simulink model "exp1_2"  (R2019a)
settings: Solver=VariableStepAuto  StartTime=0.0  StopTime=10.0  RelTol=1e-3
undefined symbols (not defined in the file or in its folder): sfunchk
settings Model: Creator=17827  LastModifiedBy=17827

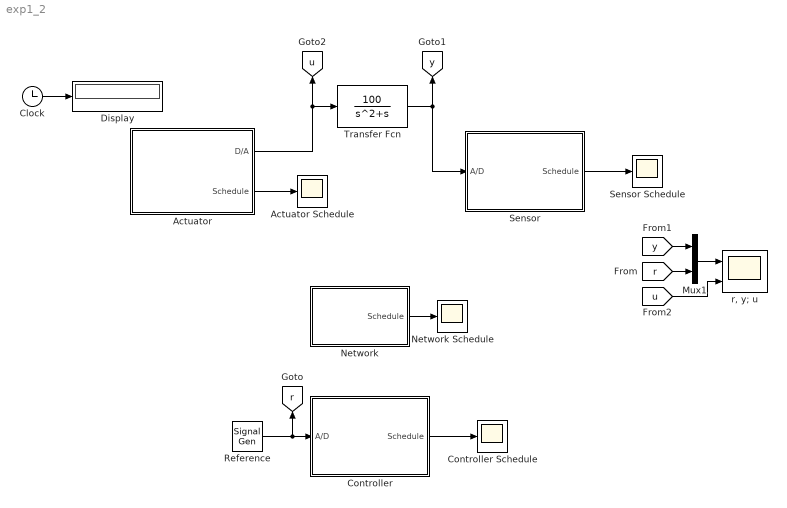
== system exp1_2 ==
  Actuator : Subsystem  AncestorBlock=truetime/TrueTime Kernel  InitFcn=sfunchk(get_param(gcb,'sfun'));  mask{sfun=actuator_init, args=[], ninputsoutputs=[0 1], ntriggers=0, trigtype=falling, nwnodenbr=3, clockoffsetdrift=[0 0], schedoutput=on, battery=off, poweroutput=off, label=1: 3}
      mask prompts: sfun "Name of init function (MEX or MATLAB):"; args "Init function argument (arbitrary struct):"; ninputsoutputs "Number of analog inputs and outputs:"; ntriggers "Number of external triggers:"; trigtype "Trigger type:"; nwnodenbr "(Network and) Node number(s):"; clockoffsetdrift "Local clock offset and drift:"; schedoutput "Show Schedule output port"; battery "Show Energy supply input port"; poweroutput "Show Power consumption output port"
      mask init:
      | ttkernel_callback(gcb,{sfun,args,ninputsoutputs,ntriggers,trigtype,nwnodenbr,clockoffsetdrift,schedoutput,battery,poweroutput})
      settings: ErrorFcn=ttkernel_error
      mask TypeOptions trigtype: rising | falling | either
      mask Display: disp(get_param(gcb,'label'))
  Actuator Schedule : Scope
  Clock : Clock
  Controller : Subsystem  AncestorBlock=truetime/TrueTime Kernel  InitFcn=sfunchk(get_param(gcb,'sfun'));  mask{sfun=controller_init, args=[], ninputsoutputs=[1 0], ntriggers=0, trigtype=falling, nwnodenbr=2, clockoffsetdrift=[0 0], schedoutput=on, battery=off, poweroutput=off, label=1: 2}
      mask prompts: sfun "Name of init function (MEX or MATLAB):"; args "Init function argument (arbitrary struct):"; ninputsoutputs "Number of analog inputs and outputs:"; ntriggers "Number of external triggers:"; trigtype "Trigger type:"; nwnodenbr "(Network and) Node number(s):"; clockoffsetdrift "Local clock offset and drift:"; schedoutput "Show Schedule output port"; battery "Show Energy supply input port"; poweroutput "Show Power consumption output port"
      mask init:
      | ttkernel_callback(gcb,{sfun,args,ninputsoutputs,ntriggers,trigtype,nwnodenbr,clockoffsetdrift,schedoutput,battery,poweroutput})
      settings: ErrorFcn=ttkernel_error
      mask TypeOptions trigtype: rising | falling | either
      mask Display: disp(get_param(gcb,'label'))
  Controller Schedule : Scope
  Display : Display
  Mux1 : Mux  Inputs=2
  Network : Subsystem  AncestorBlock=truetime/TrueTime Network  mask(Real-Time Network){nwtype=CSMA/CD (Ethernet), nwnbr=1, nnodes=3, rate=80, minsize=512, lossprob=0, seed=0, bandwidths=[0.5 0.5], slotsize=512, schedule=[1 1 2], memsize=80000, buftype=Common buffer, overflow=Retransmit, dynSchedule=0, miniSlotSize=0, NIT=0, QSortMode=FIFO, sync=0, irtSchedule=0, nrtLength=0, nodeGraph=0, scheduleoutput=on}
      mask prompts: nwtype "Network type:"; nwnbr "Network number:"; nnodes "Number of nodes:"; rate "Data rate (bits/s):"; minsize "Minimum frame size (bits):"; lossprob "Loss probability (0-1):"; seed "Initial seed:"; bandwidths "Bandwidth allocations:"; slotsize "Slotsize (bits):"; schedule "Static schedule:"; memsize "Total switch memory (bits):"; buftype "Switch buffer type:"; overflow "Switch overflow behavior:"; dynSchedule "Dynamic Schedule:"; miniSlotSize "Mini slot size (bits):"; NIT "Network idle time (bits):"; QSortMode "Input Queue Sorted by:"; sync "Synchronization length (bits):"; irtSchedule "IRT Schedule [msgID from to start arrival]:"; nrtLength "RT Class 1/NRT length (bits):"; nodeGraph "Node connection graph (nbrOfnodes x nbrOfNodes):"; scheduleoutput "Show Schedule output port:"
      mask init:
      | ttnetwork_callback(gcb,nwnbr,nnodes,scheduleoutput)
      mask TypeOptions nwtype: CSMA/CD (Ethernet) | CSMA/AMP (CAN) | Round Robin | FDMA | TDMA | Switched Ethernet | FlexRay | PROFINET | NCM
      mask Callback nwtype: ttnetwork_callback
      mask TypeOptions buftype: Common buffer | Symmetric output buffers
      mask TypeOptions overflow: Retransmit | Drop
      mask TypeOptions QSortMode: FIFO | Priority
      mask Display: disp(nwnbr)
  Network Schedule : Scope
  Reference : SignalGenerator  WaveForm=square
  Sensor : Subsystem  AncestorBlock=truetime/TrueTime Kernel  InitFcn=sfunchk(get_param(gcb,'sfun'));  mask{sfun=sensor_init, args=[], ninputsoutputs=[1 0], ntriggers=0, trigtype=falling, nwnodenbr=1, clockoffsetdrift=[0 0], schedoutput=on, battery=off, poweroutput=off, label=1: 1}
      mask prompts: sfun "Name of init function (MEX or MATLAB):"; args "Init function argument (arbitrary struct):"; ninputsoutputs "Number of analog inputs and outputs:"; ntriggers "Number of external triggers:"; trigtype "Trigger type:"; nwnodenbr "(Network and) Node number(s):"; clockoffsetdrift "Local clock offset and drift:"; schedoutput "Show Schedule output port"; battery "Show Energy supply input port"; poweroutput "Show Power consumption output port"
      mask init:
      | ttkernel_callback(gcb,{sfun,args,ninputsoutputs,ntriggers,trigtype,nwnodenbr,clockoffsetdrift,schedoutput,battery,poweroutput})
      settings: ErrorFcn=ttkernel_error
      mask TypeOptions trigtype: rising | falling | either
      mask Display: disp(get_param(gcb,'label'))
  Sensor Schedule : Scope
  Transfer Fcn : TransferFcn  Numerator=[100]  Denominator=[1 1 0]
  "r, y; u" : Scope  NumInputPorts=2
  tag scope: r=global, u=global, y=global
  wires:
  Actuator/1(D/A) -> [u], Transfer Fcn/1
  Transfer Fcn/1 -> Sensor/1(A/D), [y]
  Reference/1 -> Controller/1(A/D), [r]
  Clock/1 -> Display/1
  Mux1/1 -> "r, y; u"/1
  [r] -> Mux1/2
  [u] -> "r, y; u"/2
  [y] -> Mux1/1
  Network/1(Schedule) -> Network Schedule/1
  Controller/1(Schedule) -> Controller Schedule/1
  Actuator/2(Schedule) -> Actuator Schedule/1
  Sensor/1(Schedule) -> Sensor Schedule/1

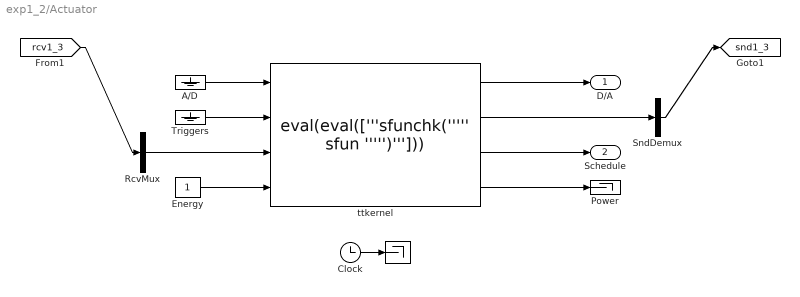
== system exp1_2/Actuator ==
  " " : Terminator
  A/D : Ground
  Clock : Clock
  Energy : Constant
  Power : Terminator
  RcvMux : Mux  Inputs=1
  SndDemux : Demux  Outputs=1
  Triggers : Ground
  ttkernel : S-Function  FunctionName=eval(eval(['''sfunchk(''''' sfun ''''')''']))  Parameters=sfun, args, ninputsoutputs, ntriggers, trigtype, nwnodenbr, clockoffsetdrift  SFunctionDeploymentMode=off  EnableBusSupport=off
  D/A : Outport
  Schedule : Outport  Port=2
  tag scope: snd1_3=global
  wires:
  Clock/1 -> " "/1
  RcvMux/1 -> ttkernel/3
  Triggers/1 -> ttkernel/2
  ttkernel/3 -> Schedule/1
  ttkernel/1 -> D/A/1
  ttkernel/2 -> SndDemux/1
  A/D/1 -> ttkernel/1
  Energy/1 -> ttkernel/4
  ttkernel/4 -> Power/1
  [rcv1_3] -> RcvMux/1
  SndDemux/1 -> [snd1_3]

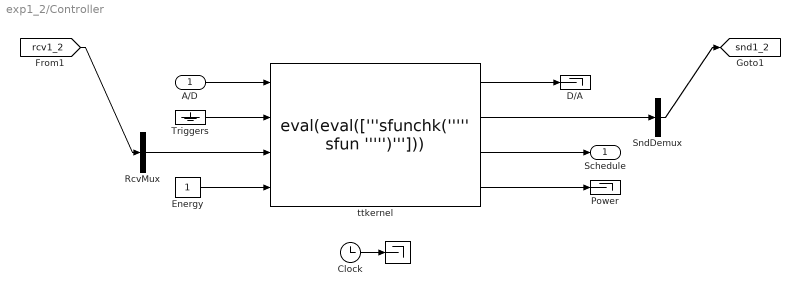
== system exp1_2/Controller ==
  A/D : Inport
  " " : Terminator
  Clock : Clock
  D/A : Terminator
  Energy : Constant
  Power : Terminator
  RcvMux : Mux  Inputs=1
  SndDemux : Demux  Outputs=1
  Triggers : Ground
  ttkernel : S-Function  FunctionName=eval(eval(['''sfunchk(''''' sfun ''''')''']))  Parameters=sfun, args, ninputsoutputs, ntriggers, trigtype, nwnodenbr, clockoffsetdrift  SFunctionDeploymentMode=off  EnableBusSupport=off
  Schedule : Outport
  tag scope: snd1_2=global
  wires:
  Clock/1 -> " "/1
  RcvMux/1 -> ttkernel/3
  Triggers/1 -> ttkernel/2
  ttkernel/3 -> Schedule/1
  ttkernel/2 -> SndDemux/1
  A/D/1 -> ttkernel/1
  Energy/1 -> ttkernel/4
  ttkernel/4 -> Power/1
  ttkernel/1 -> D/A/1
  [rcv1_2] -> RcvMux/1
  SndDemux/1 -> [snd1_2]

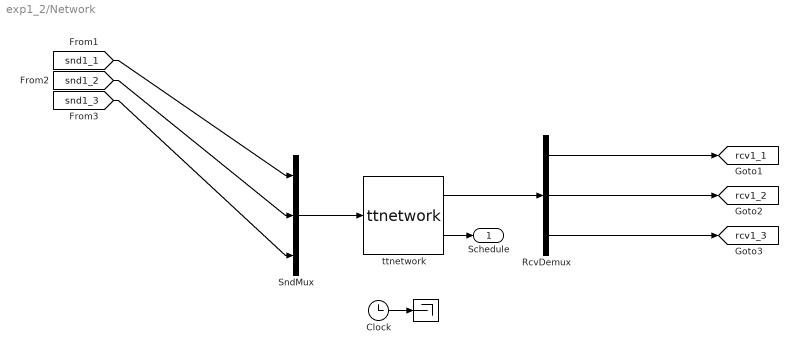
== system exp1_2/Network ==
  " " : Terminator
  Clock : Clock
  RcvDemux : Demux  Outputs=3
  SndMux : Mux  Inputs=3
  ttnetwork : S-Function  FunctionName=ttnetwork  Parameters=nwtype,nwnbr,nnodes,rate,minsize,lossprob,bandwidths,slotsize,schedule,memsize,buftype,overflow,seed,dynSchedule,miniSlotSize,NIT,QSortMode,sync,irtSchedule,nrtLength,nodeGraph  SFunctionDeploymentMode=off  EnableBusSupport=off
  Schedule : Outport
  tag scope: rcv1_1=global, rcv1_2=global, rcv1_3=global
  wires:
  Clock/1 -> " "/1
  SndMux/1 -> ttnetwork/1
  ttnetwork/1 -> RcvDemux/1
  ttnetwork/2 -> Schedule/1
  [snd1_1] -> SndMux/1
  [snd1_2] -> SndMux/2
  [snd1_3] -> SndMux/3
  RcvDemux/1 -> [rcv1_1]
  RcvDemux/2 -> [rcv1_2]
  RcvDemux/3 -> [rcv1_3]

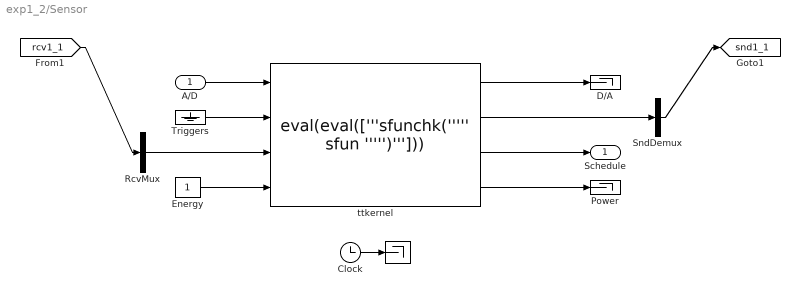
== system exp1_2/Sensor ==
  A/D : Inport
  " " : Terminator
  Clock : Clock
  D/A : Terminator
  Energy : Constant
  Power : Terminator
  RcvMux : Mux  Inputs=1
  SndDemux : Demux  Outputs=1
  Triggers : Ground
  ttkernel : S-Function  FunctionName=eval(eval(['''sfunchk(''''' sfun ''''')''']))  Parameters=sfun, args, ninputsoutputs, ntriggers, trigtype, nwnodenbr, clockoffsetdrift  SFunctionDeploymentMode=off  EnableBusSupport=off
  Schedule : Outport
  tag scope: snd1_1=global
  wires:
  Clock/1 -> " "/1
  RcvMux/1 -> ttkernel/3
  ttkernel/3 -> Schedule/1
  ttkernel/1 -> D/A/1
  ttkernel/2 -> SndDemux/1
  A/D/1 -> ttkernel/1
  Energy/1 -> ttkernel/4
  ttkernel/4 -> Power/1
  Triggers/1 -> ttkernel/2
  [rcv1_1] -> RcvMux/1
  SndDemux/1 -> [snd1_1]
